simulink model "rtwdemo_tflblas"  (Simulink 7.6)
settings: Solver=FixedStepDiscrete  StartTime=0.0  StopTime=20  FixedStep=.01  RelTol=1e-3  SampleTimeConstraint=Specified
PreLoadFcn:
  | addpath(fullfile(matlabroot,'toolbox','rtw','rtwdemos','tfl_demo'));
  | sl_refresh_customizations;
libraries: rtwdemowidgets x2
settings Model: Creator=The MathWorks Inc.  ExtModeAutoUpdateStatusClock=off
settings MATStruct: SampleTime=1  Offset=0  Priority=[30.0]
settings DataIOCC: SaveOutput=off  SaveTime=off  SignalLoggingName=sigsOut
settings OptimizationCC: InlineParams=on  UseIntDivNetSlope=on  InlineInvariantSignals=on  EnhancedBackFolding=on  BooleansAsBitfields=on  PassReuseOutputArgsAs=Individual arguments  StateBitsets=on  DataBitsets=on  UseTempVars=on  ZeroExternalMemoryAtStartup=off  ZeroInternalMemoryAtStartup=off  NoFixptDivByZeroProtection=on  EfficientFloat2IntCast=on  OptimizeModelRefInitCode=on  LifeSpan=1
settings DebuggingCC: CheckExecutionContextPreStartOutputMsg=on  CheckExecutionContextRuntimeOutputMsg=on  SolverPrmCheckMsg=none  IntegerOverflowMsg=none  StrictBusMsg=ErrorOnBusTreatedAsVector
settings HardwareCC: ProdBitPerLong=64  ProdIntDivRoundTo=Zero  ProdEndianess=LittleEndian  ProdWordSize=64  ProdHWDeviceType=Specified  TargetHWDeviceType=32-bit Generic
settings SFSimCC: SFSimEnableDebug=off  SFSimOverflowDetection=off  SimParseCustomCode=off
settings RTWCC: SystemTargetFile=ert.tlc  TemplateMakefile=ert_default_tmf  Description=Real-Time Workshop Embedded Coder  GenerateReport=on  RTWVerbose=off  ProcessScript=ert_make_rtw_hook  IncludeHyperlinkInReport=on  LaunchReport=on  GenerateTraceInfo=on  GenerateTraceReport=on  GenerateTraceReportSl=on  GenerateTraceReportSf=on  GenerateTraceReportEml=on
settings CodeAppCC: ForceParamTrailComments=on  IgnoreCustomStorageClasses=off  IgnoreTestpoints=on  SimulinkDataObjDesc=on  CustomSymbolStrGlobalVar=rt$N$M  CustomSymbolStrType=$N$M  CustomSymbolStrFcn=$N$M$F  CustomSymbolStrMacro=$N$M  InsertBlockDesc=on
settings ERTTargetCC: TargetFunctionLibrary=Matrix Multiplication to BLAS Examples  MultiwordLength=2048  GenerateSampleERTMain=on  IncludeMdlTerminateFcn=off  SupportNonFinite=off  InlinedParameterPlacement=NonHierarchical  ERTCustomFileTemplate=example_file_process.tlc  ConvertIfToSwitch=off

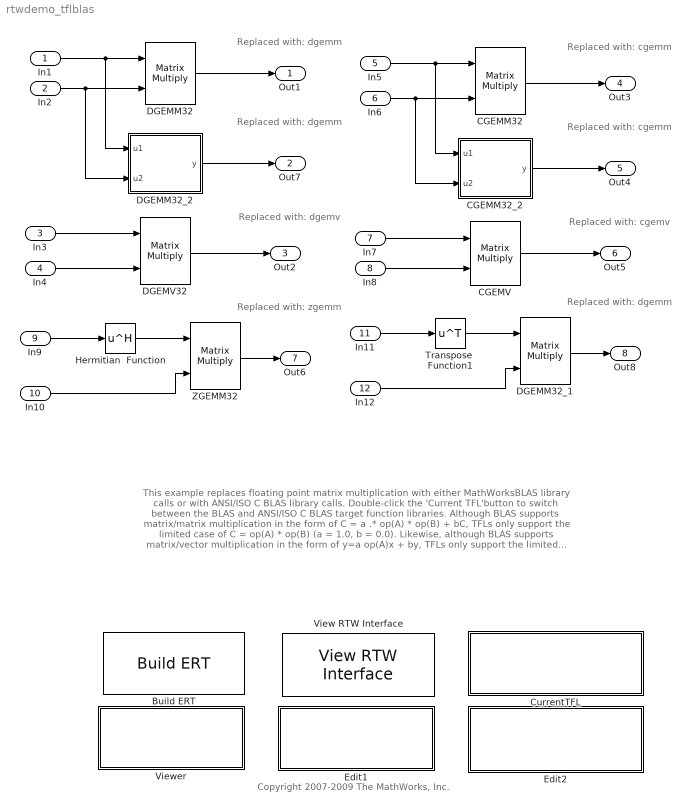
== system rtwdemo_tflblas ==
  note: Copyright 2007-2009 The MathWorks, Inc.
  note: Replaced with:
      | dgemm
  note: Replaced with:
      | dgemm
  note: Replaced with:
      | dgemv
  note: Replaced with:
      | cgemm
  note: Replaced with:
      | cgemm
  note: Replaced with:
      | cgemv
  note: Replaced with:
      | zgemm
  note: Replaced with:
      | dgemm
  note: This example replaces floating point matrix multiplication with either MathWorksBLAS library calls or with ANSI/ISO C BLAS library calls.
      | Double-click the 'Current TFL'button to switch between the BLAS  and ANSI/ISO C BLAS target function libraries.
      |
      | Although BLAS supports matrix/matrix multiplication in the form of C = a .* op(A) * op(B) + bC,
      | TFLs only support the limited case of C = op(A) * op(B) (a = 1.0, b = 0.0).
      | Likewise, although BLAS supports matrix/vector multiplication in the form of y=a op(A)x + by,
      | TFLs only support the limited case of y = op(A) x (a = 1.0, b = 0.0)
      | Here, op(X) = X (no Transpose), XT (Transpose), XH(Conjugate Transpose)
      |
      | The MathWorks BLAS library is supported on Windows and UNIX platforms.
      |
      | The C BLAS example does not include BLAS implementations and
      | therefore does not create an executable.
  In1 : Inport  OutDataTypeStr=double  PortDimensions=[10 20]  SampleTime=1
  In2 : Inport  Port=2  OutDataTypeStr=double  PortDimensions=[20 10]  SampleTime=1
  In3 : Inport  Port=3  OutDataTypeStr=double  PortDimensions=[10 20]  SampleTime=1
  In4 : Inport  Port=4  OutDataTypeStr=double  PortDimensions=[20 1]  SampleTime=1
  In5 : Inport  Port=5  OutDataTypeStr=single  PortDimensions=[10 20]  SampleTime=1
      settings: SignalType=complex
  In6 : Inport  Port=6  OutDataTypeStr=single  PortDimensions=[20 10]  SampleTime=1
      settings: SignalType=complex
  In7 : Inport  Port=7  OutDataTypeStr=single  PortDimensions=[10 20]  SampleTime=1
      settings: SignalType=complex
  In8 : Inport  Port=8  OutDataTypeStr=single  PortDimensions=[20 1]  SampleTime=1
      settings: SignalType=complex
  In9 : Inport  Port=9  OutDataTypeStr=double  PortDimensions=[10 10]  SampleTime=1
      settings: SignalType=complex
  In10 : Inport  Port=10  OutDataTypeStr=double  PortDimensions=[10 10]  SampleTime=1
      settings: SignalType=complex
  In11 : Inport  Port=11  OutDataTypeStr=double  PortDimensions=[10 10]  SampleTime=1
  In12 : Inport  Port=12  OutDataTypeStr=double  PortDimensions=[10 10]  SampleTime=1
  Build ERT : rtwdemowidgets/Build ERT  SystemSampleTime=-1  attrib_overrides={'GenFloatMathFcnCalls', 'SupportComplex','GenCodeOnly'}
  CGEMM32 : Product  Multiplication=Matrix(*)  OutDataTypeStr=single  SaturateOnIntegerOverflow=on  RndMeth=Zero
  CGEMM32_2 : Stateflow chart  TreatAsAtomicUnit=on
  CGEMV : Product  Multiplication=Matrix(*)  OutDataTypeStr=single  SaturateOnIntegerOverflow=on  RndMeth=Zero
  CurrentTFL : Subsystem  mask{tflName=BLAS}
      mask prompts: tflName "Name"
      mask help: Enter the attributes of the configuration set that you want preserved. Otherwise, the default configuration script will override your current settings.
      settings: OpenFcn=|
      | tfl = get_param(gcs,'TargetFunctionLibrary');
      | if strcmp(tfl,'Matrix Multiplication to BLAS Examples')                                           set_param(gcs,'TargetFunctionLibrary', 'Matrix Multiplication to C BLAS Examples');
      | set_param(gcs,'GenCodeOnly','on');    set_param(gcb,'MaskValues',{'C BLAS'});
      | 
      | else
      | set_param(gcs,'TargetFunctionLibrary', 'Matrix Multiplication to BLAS Examples');
      | set_param(gcs','GenCodeOnly','off');    set_param(gcb,'MaskValues',{'BLAS'});
      | 
      | end
      | clear tfl;
      mask Display: disp(['Current TFL: ',tflName,'\n(double-click to swap)'])
  DGEMM32 : Product  Multiplication=Matrix(*)  OutDataTypeStr=double  SaturateOnIntegerOverflow=on  RndMeth=Zero
  DGEMM32_1 : Product  Multiplication=Matrix(*)  OutDataTypeStr=double  SaturateOnIntegerOverflow=on  RndMeth=Zero
  DGEMM32_2 : Stateflow chart  TreatAsAtomicUnit=on
  DGEMV32 : Product  Multiplication=Matrix(*)  OutDataTypeStr=double  SaturateOnIntegerOverflow=on  RndMeth=Zero
  Edit1 : Subsystem  mask{attrib_overrides={}}
      mask prompts: attrib_overrides "List of attributes to preserve (cell of strings):"
      mask help: Enter the attributes of the configuration set that you want preserved. Otherwise, the default configuration script will override your current settings.
      settings: OpenFcn=|
      | edit('tfl_table_tmwblas');
      | edit('tfl_table_cblas');
      mask Display:
      | disp(['View/edit TFL\n',...
      | 	  'Definition Files\n(double-click)'])
  Edit2 : Subsystem  mask{attrib_overrides={}}
      mask prompts: attrib_overrides "List of attributes to preserve (cell of strings):"
      mask help: Enter the attributes of the configuration set that you want preserved. Otherwise, the default configuration script will override your current settings.
      settings: OpenFcn=edit(fullfile(matlabroot,'toolbox','rtw','rtwdemos','tfl_demo', 'sl_customization.m'));
      mask Display:
      | disp(['View/edit TFL Registration\n',...
      | 	  'sl_customization.m\n(double-click)'])
  Hermitian  Function : Math  Operator=hermitian  SaturateOnIntegerOverflow=on
  Transpose  Function1 : Math  Operator=transpose  SaturateOnIntegerOverflow=on
  View RTW Interface : rtwdemowidgets/View RTW Interface  SystemSampleTime=-1
  Viewer : Subsystem  mask{attrib_overrides={}}
      mask prompts: attrib_overrides "List of attributes to preserve (cell of strings):"
      mask help: Enter the attributes of the configuration set that you want preserved. Otherwise, the default configuration script will override your current settings.
      settings: OpenFcn=|
      | tfl = get_param(gcs,'TargetFunctionLibrary');
      | if strcmp(tfl,'Matrix Multiplication to BLAS Examples')
      | h = tfl_table_tmwblas
      | else
      | h = tfl_table_cblas
      | end
      | obj = RTW.viewTfl(h);
      | clear tfl obj h;
      mask Display:
      | disp(['Invoke TFL Viewer on\n',...
      | 	  'Currently Selected TFL\n(double-click)'])
  ZGEMM32 : Product  Multiplication=Matrix(*)  OutDataTypeStr=double  SaturateOnIntegerOverflow=on  RndMeth=Zero
  Out1 : Outport
  Out7 : Outport  Port=2
  Out2 : Outport  Port=3
  Out3 : Outport  Port=4
  Out4 : Outport  Port=5
  Out5 : Outport  Port=6
  Out6 : Outport  Port=7
  Out8 : Outport  Port=8
  wires:
  DGEMM32/1 -> Out1/1
  In1/1 -> DGEMM32/1, DGEMM32_2/1(u1)
  In2/1 -> DGEMM32/2, DGEMM32_2/2(u2)
  DGEMM32_2/1(y) -> Out7/1
  DGEMV32/1 -> Out2/1
  In3/1 -> DGEMV32/1
  In4/1 -> DGEMV32/2
  CGEMM32/1 -> Out3/1
  In5/1 -> CGEMM32_2/1(u1), CGEMM32/1
  In6/1 -> CGEMM32_2/2(u2), CGEMM32/2
  CGEMM32_2/1(y) -> Out4/1
  CGEMV/1 -> Out5/1
  In7/1 -> CGEMV/1
  In8/1 -> CGEMV/2
  ZGEMM32/1 -> Out6/1
  In9/1 -> Hermitian  Function/1
  In10/1 -> ZGEMM32/2
  Hermitian  Function/1 -> ZGEMM32/1
  DGEMM32_1/1 -> Out8/1
  In11/1 -> Transpose  Function1/1
  In12/1 -> DGEMM32_1/2
  Transpose  Function1/1 -> DGEMM32_1/1

== system rtwdemo_tflblas/CurrentTFL ==

== system rtwdemo_tflblas/Edit1 ==

== system rtwdemo_tflblas/Edit2 ==

== system rtwdemo_tflblas/Viewer ==

== matlab function CGEMM32_2 ==
  data: u1 input uint32; y output uint32; u2 input uint32
function y = fcn(u1, u2)
% This block supports the Embedded MATLAB subset.
% See the help menu for details. 

y = u1 * u2;

== matlab function DGEMM32_2 ==
  data: u1 input uint32; y output uint32; u2 input uint32
function y = fcn(u1, u2)
% This block supports the Embedded MATLAB subset.
% See the help menu for details. 

y = u1 * u2;
